simulink library "PaperLib"  (R2025a)
settings: Solver=VariableStepAuto  StartTime=0.0  StopTime=10.0  RelTol=1e-3
libraries: StdLib x4
settings Model: Creator=peter  LastModifiedBy=peter
settings RTWCC: GPUComputeCapability=3.5

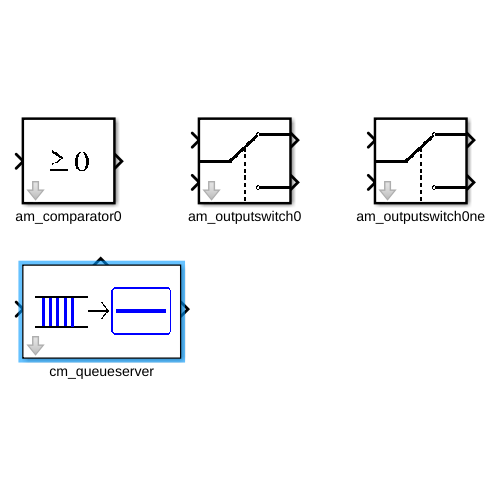
[thumbnail: Simulink's stored preview of the top-level diagram]
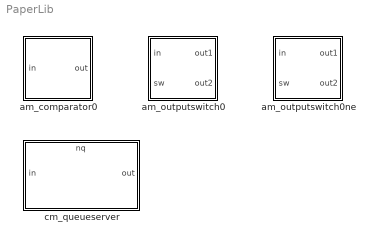
== system PaperLib ==
  am_comparator0 : Subsystem  TreatAsAtomicUnit=on  mask(Comparator){tau=[0,1], debug=0}
      mask help: Returns 1 if in >= 0, else 0.
      mask Help:
      | <p>Returns 1 if in >= 0, else 0.</p>
      | 
      | <p>Ports
      | <ul>
      | <li>inputs:
      |   <ul>
      |     <li>in: incoming value</li>
      |   </ul>
      | </li>
      | <li>outputs:
      |   <ul>
      |     <li>out: result value</li>
      |   </ul>
      | </li>
      | </ul>
      | </p>
      | 
      | <p>System Parameters
      | <ul>
      | <li>debug: flag to enable debug information</li>
      | <li>tau:   infinitesimal delay</li>
      | </ul>
      | </p>
      | 
      | <p>States
      | <ul>
      | <li>s:   running</li>
      | </ul>
      | </p>
      mask DialogControl Container6 Prompt: Advanced
      mask Display: image('icon_comparator.png');
  am_outputswitch0 : Subsystem  TreatAsAtomicUnit=on  mask(Outputswitch){port0=1, tau=[0,1], debug=0}
      mask prompts: port0 "initial output port"
      mask help: Routes input to one of two outputs according to sw input.
      mask Help:
      | <p>Routes input to one of two outputs according to sw input.</p>
      | 
      | <p>Ports
      | <ul>
      | <li>inputs:
      |   <ul>
      |     <li>in: incoming entities</li>
      |     <li>sw: output selector</li>
      |   </ul>
      | </li>
      | <li>outputs:
      |   <ul>
      |     <li>out1/2: outgoing entities</li>
      |   </ul>
      | </li>
      | </ul>
      | </p>
      | 
      | <p>System Parameters
      | <ul>
      | <li>port0:  initial output port</li>
      | <li>debug: flag to enable debug information</li>
      | <li>tau:   infinitesimal delay</li>
      | </ul>
      | </p>
      | 
      | <p>States
      | <ul>
      | <li>s:   running</li>
      | <li>nextPort:  output port of new in values</li>
      | </ul>
      | </p>
      mask DialogControl Container4 Prompt: General
      mask DialogControl Container5 Prompt: Advanced
      mask Display: image('icon_outputswitch.png');
  am_outputswitch0ne : Subsystem  TreatAsAtomicUnit=on  mask(Outputswitch){port0=1, tau=[0,1], debug=0}
      mask prompts: port0 "initial output port"
      mask help: Routes input to one of two outputs according to sw input.
      mask Help:
      | <p>Routes input to one of two outputs according to sw input.</p>
      | 
      | <p>Ports
      | <ul>
      | <li>inputs:
      |   <ul>
      |     <li>in: incoming entities</li>
      |     <li>sw: output selector</li>
      |   </ul>
      | </li>
      | <li>outputs:
      |   <ul>
      |     <li>out1/2: outgoing entities</li>
      |   </ul>
      | </li>
      | </ul>
      | </p>
      | 
      | <p>System Parameters
      | <ul>
      | <li>port0:  initial output port</li>
      | <li>debug: flag to enable debug information</li>
      | <li>tau:   infinitesimal delay</li>
      | </ul>
      | </p>
      | 
      | <p>States
      | <ul>
      | <li>s:   running</li>
      | <li>nextPort:  output port of new in values</li>
      | </ul>
      | </p>
      mask DialogControl Container4 Prompt: General
      mask DialogControl Container5 Prompt: Advanced
      mask Display: image('icon_outputswitch.png');
  cm_queueserver : Subsystem  mask{ts=4.5, tau=[0,1], debug=0}
      settings: PortSchema="{\"entries\":[{\"content\":{\"sides\":[{\"content\":{\"connectorIds\":[\"In1\"]},\"type\":\"ConnectorPlacement.EquallySpacedRectSide\",\"uuid\":\"07fa0e51-8843-4ac9-8e94-884ae9a89d36\"},{\"content\":{\"connectorIds\":[\"Out1\"],\"side\":\"RIGHT\"},\"type\":\"ConnectorPlacement.EquallySpacedRectSide\",\"uuid\":\"0131ce69-7449-4362-9cfd-88c0df269334\"},{\"content\":{\"connectorIds\":[\"Out2\"],\"side\":\"TOP\"},\"type\":\"ConnectorPlacement.EquallySpacedRectSide\",\"uuid\":\"407e2fdf-9916-4f3f-84c2-2a472bd1d59f\"}]},\"type\":\"ConnectorPlacement.EquallySpacedConnector\",\"uuid\":\"291a1c46-4425-425c-bba8-593c7bd17cc2\"}],\"packageUris\":[\"http://schema.mathworks.com/mf0/Connector/R2020b\"],\"version\":\"1.0\"}"
      mask DialogControl Container4 Prompt: General
      mask DialogControl Container5 Prompt: Advanced
      mask Display: image('icon_queueserver.png');

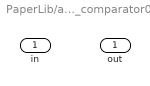
== system PaperLib/am_comparator0 ==
  in : Inport
  out : Outport

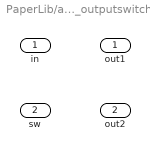
== system PaperLib/am_outputswitch0 ==
  in : Inport
  sw : Inport  Port=2
  out1 : Outport
  out2 : Outport  Port=2

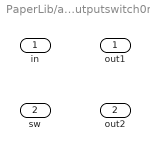
== system PaperLib/am_outputswitch0ne ==
  in : Inport
  sw : Inport  Port=2
  out1 : Outport
  out2 : Outport  Port=2

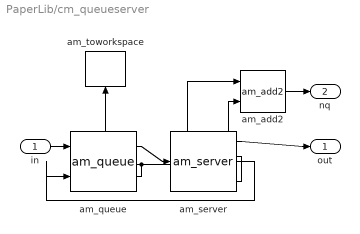
== system PaperLib/cm_queueserver ==
  in : Inport
  am_add2 : StdLib/am_add2  tau=tau  debug=debug
      settings: SourceProductName=Math Operations
  am_queue : StdLib/am_queue  tD=2*tau  tau=tau  debug=debug
      settings: SourceProductName=Logistics
  am_server : StdLib/am_server  tS=ts  tsField="\"\""  tau=tau  debug=debug
      settings: SourceProductName=Logistics
  am_toworkspace : StdLib/am_toworkspace  varname="\"nq1\""  t0=0  format="\"vector\""  tau=[0,5]  debug=0
  out : Outport
  nq : Outport  Port=2
  wires:
  am_add2/1 -> nq/1
  am_server/3 -> am_add2/2
  am_queue/2 -> am_toworkspace/1, am_add2/1
  am_server/1 -> out/1
  am_server/2 -> am_queue/2
  in/1 -> am_queue/1
  am_queue/1 -> am_server/1
